simulink model "Controle_CTC"  (R2024b)
settings: Solver=FixedStepAuto  StartTime=0.0  StopTime=10  FixedStep=.01  RelTol=1e-3
settings Model: Creator=IDRZBOOK002  LastModifiedBy=IDRZBOOK002

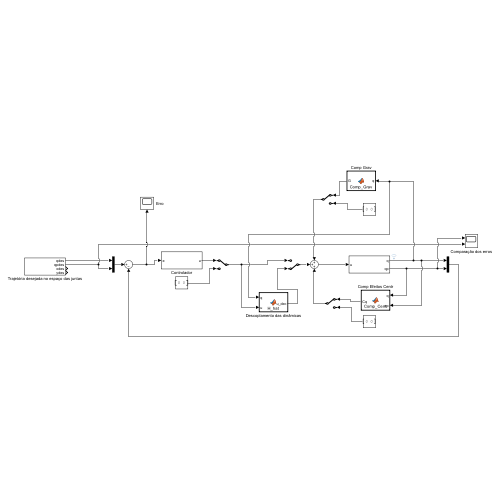
[thumbnail: Simulink's stored preview of the top-level diagram]
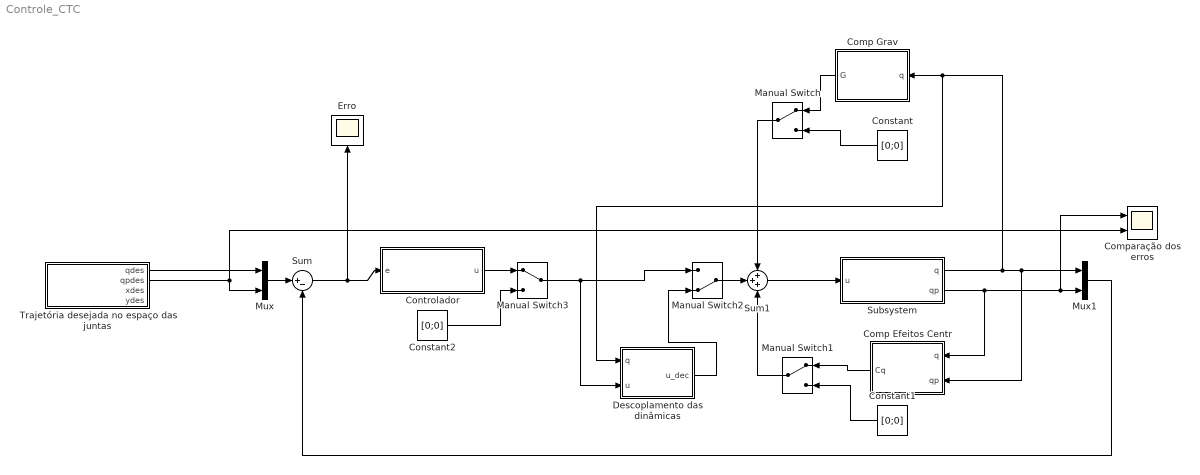
== system Controle_CTC ==
  Comp Efeitos Centr : MATLAB Function  TreatAsAtomicUnit=on
  Comp Grav : MATLAB Function  TreatAsAtomicUnit=on
  Comparação dos erros : Scope  NumInputPorts=2
  Constant : Constant  Value=[0;0]
  Constant1 : Constant  Value=[0;0]
  Constant2 : Constant  Value=[0;0]
  Controlador : Subsystem
  Descoplamento das dinâmicas : MATLAB Function  TreatAsAtomicUnit=on
  Erro : Scope
  Manual Switch : ManualSwitch
  Manual Switch1 : ManualSwitch
  Manual Switch2 : ManualSwitch  CurrentSetting=0
  Manual Switch3 : ManualSwitch
  Mux : Mux  Inputs=2
  Mux1 : Mux  Inputs=2
  Subsystem : Subsystem
  Sum : Sum  Inputs=|+-
  Sum1 : Sum  Inputs=+++
  Trajetória desejada no espaço das juntas : Subsystem
  wires:
  Trajetória desejada no espaço das juntas/1(qdes) -> Mux/1
  Trajetória desejada no espaço das juntas/2(qpdes) -> Mux/2, Comparação dos erros/2
  Mux/1 -> Sum/1
  Sum/1 -> Controlador/1(e), Erro/1
  Subsystem/1(q) -> Descoplamento das dinâmicas/1(q), Comp Grav/1(q), Comp Efeitos Centr/2(qp), Mux1/1
  Mux1/1 -> Sum/2
  Manual Switch/1 -> Sum1/1
  Sum1/1 -> Subsystem/1(u)
  Constant/1 -> Manual Switch/2
  Comp Grav/1(G) -> Manual Switch/1
  Manual Switch1/1 -> Sum1/3
  Subsystem/2(qp) -> Comp Efeitos Centr/1(q), Comparação dos erros/1, Mux1/2
  Comp Efeitos Centr/1(Cq) -> Manual Switch1/1
  Constant1/1 -> Manual Switch1/2
  Manual Switch2/1 -> Sum1/2
  Descoplamento das dinâmicas/1(u_dec) -> Manual Switch2/2
  Manual Switch3/1 -> Descoplamento das dinâmicas/2(u), Manual Switch2/1
  Controlador/1(u) -> Manual Switch3/1
  Constant2/1 -> Manual Switch3/2

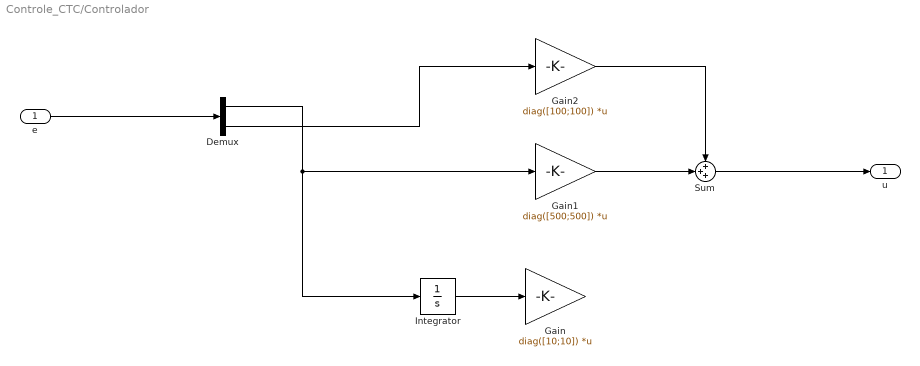
== system Controle_CTC/Controlador ==
  e : Inport
  Demux : Demux  Outputs=2
  Gain : Gain  Gain=diag([10;10])  Multiplication=Matrix(K*u) (u vector)
  Gain1 : Gain  Gain=diag([500;500])  Multiplication=Matrix(K*u) (u vector)
  Gain2 : Gain  Gain=diag([100;100])  Multiplication=Matrix(K*u) (u vector)
  Integrator : Integrator
  Sum : Sum  Inputs=+++
  u : Outport
  wires:
  Integrator/1 -> Gain/1
  Gain1/1 -> Sum/2
  Gain2/1 -> Sum/1
  e/1 -> Demux/1
  Demux/1 -> Integrator/1, Gain1/1
  Demux/2 -> Gain2/1
  Sum/1 -> u/1

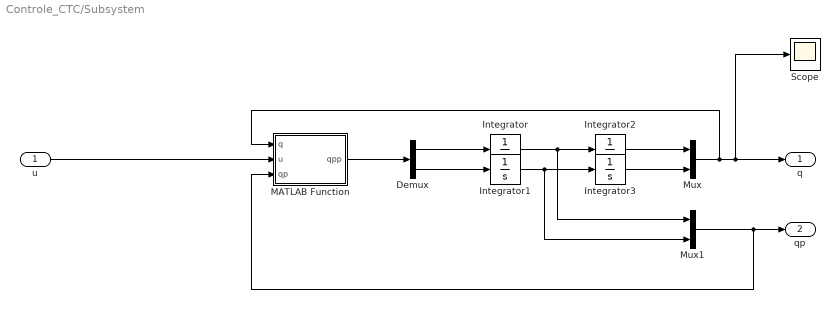
== system Controle_CTC/Subsystem ==
  u : Inport
  Demux : Demux  Outputs=2
  Integrator : Integrator
  Integrator1 : Integrator
  Integrator2 : Integrator  InitialCondition=pi/3
  Integrator3 : Integrator  InitialCondition=pi/2
  MATLAB Function : MATLAB Function  TreatAsAtomicUnit=on
  Mux : Mux  Inputs=2
  Mux1 : Mux  Inputs=2
  Scope : Scope
  q : Outport
  qp : Outport  Port=2
  wires:
  u/1 -> MATLAB Function/2(u)
  Demux/1 -> Integrator/1
  Demux/2 -> Integrator1/1
  Integrator1/1 -> Mux1/2, Integrator3/1
  Integrator2/1 -> Mux/1
  Integrator3/1 -> Mux/2
  Integrator/1 -> Mux1/1, Integrator2/1
  Mux1/1 -> MATLAB Function/3(qp), qp/1
  Mux/1 -> Scope/1, q/1, MATLAB Function/1(q)
  MATLAB Function/1(qpp) -> Demux/1

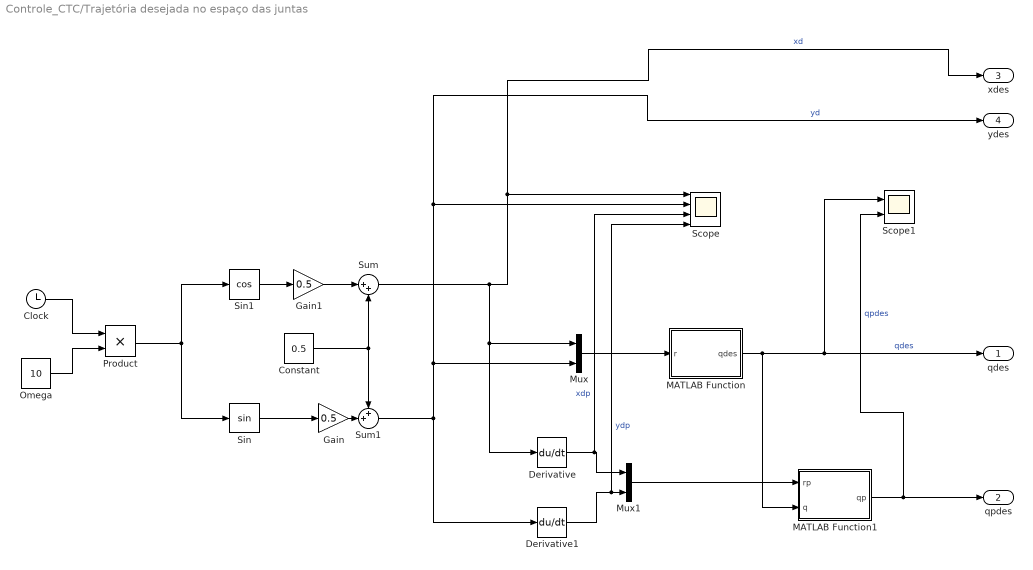
== system Controle_CTC/Trajetória desejada no espaço das juntas ==
  Clock : Clock
      settings: Decimation=100
  Constant : Constant  Value=0.5
  Derivative : Derivative
  Derivative1 : Derivative
  Gain : Gain  Gain=0.5
  Gain1 : Gain  Gain=0.5
  MATLAB Function : MATLAB Function  TreatAsAtomicUnit=on
  MATLAB Function1 : MATLAB Function  TreatAsAtomicUnit=on
  Mux : Mux  Inputs=2
  Mux1 : Mux  Inputs=2
  Omega : Constant  Value=10
  Product : Product
  Scope : Scope  NumInputPorts=4
  Scope1 : Scope  NumInputPorts=2
  Sin : Trigonometry
  Sin1 : Trigonometry  Operator=cos
  Sum : Sum  Inputs=|++
  Sum1 : Sum  Inputs=++|
  qdes : Outport
  qpdes : Outport  Port=2
  xdes : Outport  Port=3
  ydes : Outport  Port=4
  wires:
  Sin/1 -> Gain/1
  Clock/1 -> Product/1
  Omega/1 -> Product/2
  Product/1 -> Sin1/1, Sin/1
  Sin1/1 -> Gain1/1
  Derivative/1 -> Scope/3, Mux1/1  "xdp"
  Derivative1/1 -> Mux1/2, Scope/4  "ydp"
  Mux/1 -> MATLAB Function/1(r)
  MATLAB Function/1(qdes) -> MATLAB Function1/2(q), Scope1/1, qdes/1  "qdes"
  Mux1/1 -> MATLAB Function1/1(rp)
  MATLAB Function1/1(qp) -> Scope1/2, qpdes/1  "qpdes"
  Gain1/1 -> Sum/1
  Sum/1 -> Mux/1, Derivative/1, Scope/1, xdes/1  "xd"
  Constant/1 -> Sum1/1, Sum/2
  Gain/1 -> Sum1/2
  Sum1/1 -> Scope/2, ydes/1, Mux/2, Derivative1/1  "yd"

== matlab function Controle_CTC/Trajetória desejada no espaço das juntas/MATLAB Function ==
  data: r input; qdes output
function qdes = inv_kin(r)
%Função para cálculo da cinemática inversa de posição
%r -> posição desejada
%qdes ->parâmetros de junta para a posição desejada da ferramenta

%Parâmetros Geométricos
l1 = 1;
l2 = 1;

%Cinem[atica Inversa
xe = r(1);
ye = r(2);
d2 = xe^2 + ye^2;
cos_t2 = (d2 - l1^2 - l2^2) / (2 * l1 * l2);
sin_t2 = sqrt(1 - cos_t2^2);
t2 = atan2(sin_t2, cos_t2);
t1 = atan2(ye, xe) - atan2(l2 * sin(t2), l1 + l2 * cos(t2));
%Saída da função
qdes = [t1;t2];

== matlab function Controle_CTC/Subsystem/MATLAB Function ==
  data: q input; u input; qp input; qpp output size=[2 1]
function qpp  = dinamica(q,u,qp)
%Função para o cálculo da dinâmica
q  = q(:);
u  = u(:);
qp = qp(:);
%Parâmetros de inércia e geométricos
Izz1 = 1;
Izz2 = 1;
m1 = 1;
m2 = 1;
L1 = 1;
L2 = 1;
g=9.81;

%Atribuição das variáveis
th1 = q(1);
th2 = q(2);
dth1 = qp(1);
dth2 = qp(2);

%Matrizes da equação da dinâmica
H = [Izz1 + Izz2 + 0.2500*L1^2*m1 + L1^2*m2 + 0.2500*L2^2*m2 + L1*L2*m2*cos(th2), 0.2500*m2*L2^2 + 0.5000*L1*m2*cos(th2)*L2 + Izz2;
                           0.2500*m2*L2^2 + 0.5000*L1*m2*cos(th2)*L2 + Izz2,                            0.2500*m2*L2^2 + Izz2];

C = [-0.5000*L1*L2*dth2*m2*sin(th2), -0.5000*L1*L2*m2*sin(th2)*(dth1 + dth2);
      0.5000*L1*L2*dth1*m2*sin(th2),                                       0];

G = [g*m2*(0.5000*L2*cos(th1 + th2) + L1*cos(th1)) + 0.5000*L1*g*m1*cos(th1);
                                          0.5000*L2*g*m2*cos(th1 + th2)];

%Cálculo das acelerações
qpp = H\(u-C*qp-G);

== matlab function Controle_CTC/Comp Grav ==
  data: G output; q input
function G = Comp_Grav(q)

%Parâmetros de inércia e geométricos
m1 = 1;
m2 = 1;
L1 = 1;
L2 = 1;
g=9.81;

%Atribuição das variáveis
th1 = q(1);
th2 = q(2);

G = [g*m2*(0.5000*L2*cos(th1 + th2) + L1*cos(th1)) + 0.5000*L1*g*m1*cos(th1);
                                          0.5000*L2*g*m2*cos(th1 + th2)];

== matlab function Controle_CTC/Comp Efeitos Centr ==
  data: Cq output; q input; qp input
function Cq = Comp_Cent(q,qp)

%Função para o cálculo da dinâmica
q  = q(:);
qp = qp(:);
%Parâmetros de inércia e geométricos
m2 = 1;
L1 = 1;
L2 = 1;

%Atribuição das variáveis
th2 = q(2);
dth1 = qp(1);
dth2 = qp(2);

%Matrizes da equação da dinâmica
C = [-0.5000*L1*L2*dth2*m2*sin(th2), -0.5000*L1*L2*m2*sin(th2)*(dth1 + dth2);
      0.5000*L1*L2*dth1*m2*sin(th2),                                       0];

Cq = C*qp;

== matlab function Controle_CTC/Descoplamento das dinâmicas ==
  data: q input; u input; u_dec output
function u_dec = H_hat(q,u)
%Função para o cálculo da dinâmica
q  = q(:);
u  = u(:);
th2 = q(2);

%Parâmetros de inércia e geométricos
Izz1 = 1;
Izz2 = 1;
m1 = 1;
m2 = 1;
L1 = 1;
L2 = 1;

H = [Izz1 + Izz2 + 0.2500*L1^2*m1 + L1^2*m2 + 0.2500*L2^2*m2 + L1*L2*m2*cos(th2), 0.2500*m2*L2^2 + 0.5000*L1*m2*cos(th2)*L2 + Izz2;
                           0.2500*m2*L2^2 + 0.5000*L1*m2*cos(th2)*L2 + Izz2,                            0.2500*m2*L2^2 + Izz2];
u_dec= H * u;

== matlab function Controle_CTC/Trajetória desejada no espaço das juntas/MATLAB Function1 ==
  data: rp input; qp output; q input
function qp = inv_dif_kin(rp,q)
%Função para a Cinemática inversa diferencial
%rp -> velocidade desejada
%q -> parâmetro de junta
%qp -> velocidades das juntas desejada
%Parâmetros Geométricos
l1 = 1;
l2 = 1;

%Matriz Jacobiana
J = [-l1*sin(q(1))-l2*sin(q(1)+q(2)) -l2*sin(q(1)+q(2));
    l1*cos(q(1))+l2*cos(q(1)+q(2)) l2*cos(q(1)+q(2))];

%Verificação de singularidades
if det(J)==0
    warning("Pose singular")
end

%Cálculo da velocidade das juntas
qp = J^-1*rp;
